simulink model "model1v4"  (R2020b)
settings: Solver=VariableStepAuto  StartTime=0.0  StopTime=30  RelTol=1e-3
settings Model: Creator=dkravchenko  LastModifiedBy=dkravchenko

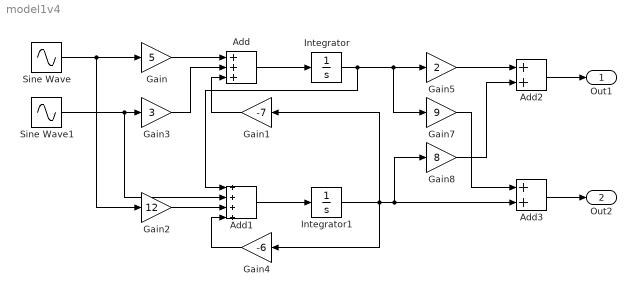
== system model1v4 ==
  Add : Sum  Inputs=+++
  Add1 : Sum  Inputs=++++
  Add2 : Sum
  Add3 : Sum
  Gain : Gain  Gain=5
  Gain1 : Gain  Gain=-7
  Gain2 : Gain  Gain=12
  Gain3 : Gain  Gain=3
  Gain4 : Gain  Gain=-6
  Gain5 : Gain  Gain=2
  Gain7 : Gain  Gain=9
  Gain8 : Gain  Gain=8
  Integrator : Integrator
  Integrator1 : Integrator
  Sine Wave : Sin  Amplitude=0  Bias=1  SampleTime=0
  Sine Wave1 : Sin  Amplitude=2  SampleTime=0
  Out1 : Outport
  Out2 : Outport  Port=2
  wires:
  Sine Wave/1 -> Gain2/1, Gain/1
  Sine Wave1/1 -> Gain3/1, Add1/2
  Gain2/1 -> Add1/3
  Gain/1 -> Add/1
  Gain3/1 -> Add/2
  Add/1 -> Integrator/1
  Add1/1 -> Integrator1/1
  Integrator1/1 -> Add3/2, Gain8/1, Gain4/1, Gain1/1
  Gain1/1 -> Add/3
  Gain4/1 -> Add1/4
  Integrator/1 -> Gain7/1, Gain5/1, Add1/1
  Gain5/1 -> Add2/1
  Gain8/1 -> Add2/2
  Gain7/1 -> Add3/1
  Add2/1 -> Out1/1
  Add3/1 -> Out2/1
